simulink model "ad_reusecode"  (R2015b)
settings: Solver=FixedStepDiscrete  SolverMode=SingleTasking  StartTime=0.0  StopTime=3  RelTol=1e-3
settings Model: Creator=at-mt  LastModifiedBy=amatsumo
settings DataIOCC: SaveFormat=Array  SignalLoggingSaveFormat=ModelDataLogs  SaveOutput=off  SignalLogging=off  SaveTime=off
settings OptimizationCC: BlockReduction=off  ConditionallyExecuteInputs=off  DefaultParameterBehavior=Inlined  ExpressionDepthLimit=2147483647
settings DebuggingCC: AlgebraicLoopMsg=error  UnderspecifiedInitializationDetection=Classic  MergeDetectMultiDrivingBlocksExec=none  SolverPrmCheckMsg=warning  SingleTaskRateTransMsg=error  FcnCallInpInsideContextMsg=UseLocalSettings  StateNameClashWarn=warning
settings HardwareCC: ProdBitPerPointer=32  ProdLargestAtomicFloat=None  ProdIntDivRoundTo=Undefined  ProdEndianess=Unspecified  ProdWordSize=32  ProdHWDeviceType=ASIC/FPGA->ASIC/FPGA  ProdEqTarget=off
settings SFSimCC: SFSimEcho=off
settings GRTTargetCC: GeneratePreprocessorConditionals=Disable all  CombineOutputUpdateFcns=off  GRTInterface=on
settings ConfigComp: CovModelRefEnable=Off  CovSFcnEnable=off

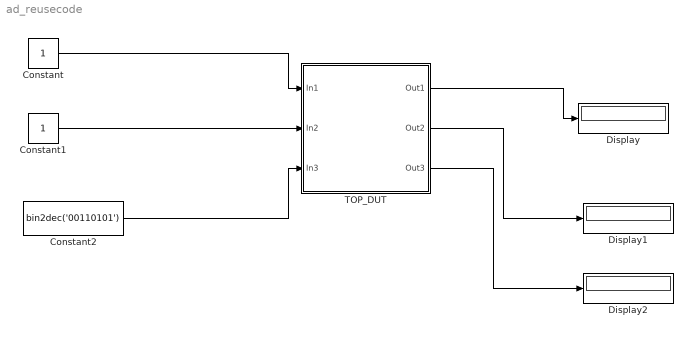
== system ad_reusecode ==
  Constant : Constant  OutDataTypeStr=boolean
  Constant1 : Constant  OutDataTypeStr=int8
  Constant2 : Constant  Value=bin2dec('00110101')  OutDataTypeStr=int8
  Display : Display
  Display1 : Display
  Display2 : Display
  TOP_DUT : Subsystem
  wires:
  TOP_DUT/1(Out1) -> Display/1
  TOP_DUT/2(Out2) -> Display1/1
  Constant/1 -> TOP_DUT/1(In1)
  Constant1/1 -> TOP_DUT/2(In2)
  Constant2/1 -> TOP_DUT/3(In3)
  TOP_DUT/3(Out3) -> Display2/1

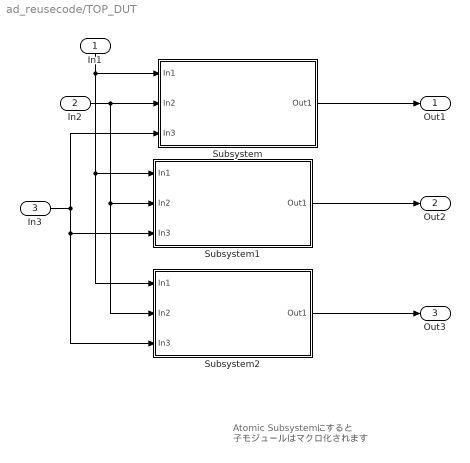
== system ad_reusecode/TOP_DUT ==
  note: Atomic Subsystemにすると
      | 子モジュールはマクロ化されます
  In1 : Inport
  In2 : Inport  Port=2
  In3 : Inport  Port=3
  Subsystem : Subsystem  TreatAsAtomicUnit=on
  Subsystem1 : Subsystem  TreatAsAtomicUnit=on
  Subsystem2 : Subsystem  TreatAsAtomicUnit=on
  Out1 : Outport
  Out2 : Outport  Port=2
  Out3 : Outport  Port=3
  wires:
  In1/1 -> Subsystem/1(In1), Subsystem1/1(In1), Subsystem2/1(In1)
  In2/1 -> Subsystem/2(In2), Subsystem1/2(In2), Subsystem2/2(In2)
  In3/1 -> Subsystem/3(In3), Subsystem1/3(In3), Subsystem2/3(In3)
  Subsystem/1(Out1) -> Out1/1
  Subsystem1/1(Out1) -> Out2/1
  Subsystem2/1(Out1) -> Out3/1

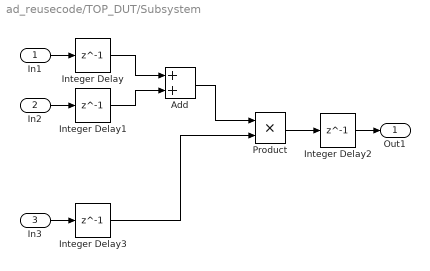
== system ad_reusecode/TOP_DUT/Subsystem ==
  In1 : Inport
  In2 : Inport  Port=2
  In3 : Inport  Port=3
  Add : Sum
  Integer Delay{,1..3} (4 alike) : Delay  DelayLength=1  InputProcessing=Inherited
  Product : Product  RndMeth=Zero
  Out1 : Outport
  wires:
  Integer Delay/1 -> Add/1
  Integer Delay1/1 -> Add/2
  Add/1 -> Product/1
  Product/1 -> Integer Delay2/1
  Integer Delay3/1 -> Product/2
  In1/1 -> Integer Delay/1
  In2/1 -> Integer Delay1/1
  Integer Delay2/1 -> Out1/1
  In3/1 -> Integer Delay3/1

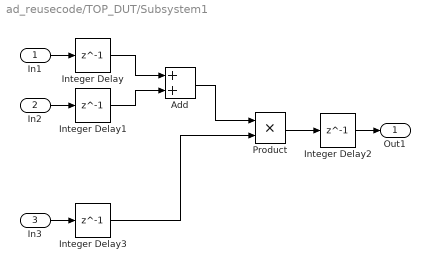
== system ad_reusecode/TOP_DUT/Subsystem1 ==
  In1 : Inport
  In2 : Inport  Port=2
  In3 : Inport  Port=3
  Add : Sum
  Integer Delay{,1..3} (4 alike) : Delay  DelayLength=1  InputProcessing=Inherited
  Product : Product  RndMeth=Zero
  Out1 : Outport
  wires:
  In3/1 -> Integer Delay3/1
  Integer Delay2/1 -> Out1/1
  In2/1 -> Integer Delay1/1
  In1/1 -> Integer Delay/1
  Integer Delay3/1 -> Product/2
  Product/1 -> Integer Delay2/1
  Add/1 -> Product/1
  Integer Delay1/1 -> Add/2
  Integer Delay/1 -> Add/1

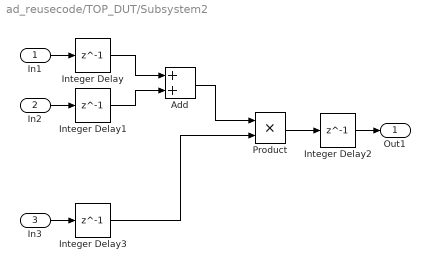
== system ad_reusecode/TOP_DUT/Subsystem2 ==
  In1 : Inport
  In2 : Inport  Port=2
  In3 : Inport  Port=3
  Add : Sum
  Integer Delay{,1..3} (4 alike) : Delay  DelayLength=1  InputProcessing=Inherited
  Product : Product  RndMeth=Zero
  Out1 : Outport
  wires:
  Integer Delay/1 -> Add/1
  Integer Delay1/1 -> Add/2
  Add/1 -> Product/1
  Product/1 -> Integer Delay2/1
  Integer Delay3/1 -> Product/2
  In1/1 -> Integer Delay/1
  In2/1 -> Integer Delay1/1
  Integer Delay2/1 -> Out1/1
  In3/1 -> Integer Delay3/1
